simulink model "practica5_simulink"  (R2024b)
settings: Solver=VariableStepAuto  StartTime=0.0  StopTime=0.01  RelTol=1e-3

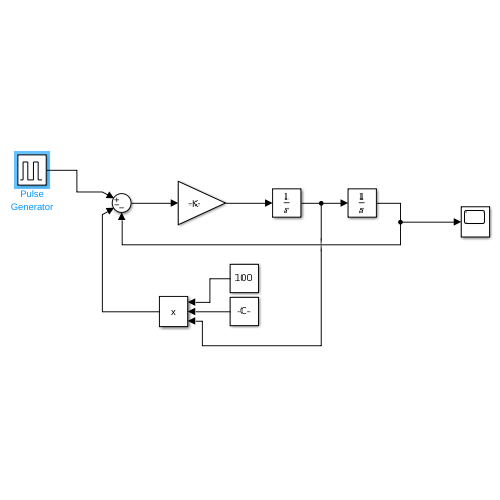
[thumbnail: Simulink's stored preview of the top-level diagram]
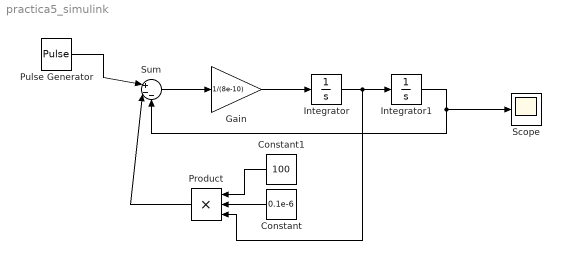
== system practica5_simulink ==
  Constant : Constant  Value=0.1e-6
  Constant1 : Constant  Value=100
  Gain : Gain  Gain=1/(8e-10)
  Integrator : Integrator
  Integrator1 : Integrator
  Product : Product  Inputs=3
  Pulse Generator : DiscretePulseGenerator  PulseType=Time based  Period=0.002  PulseWidth=50
  Scope : Scope
  Sum : Sum  Inputs=|+--
  wires:
  Integrator/1 -> Product/3, Integrator1/1
  Sum/1 -> Gain/1
  Pulse Generator/1 -> Sum/1
  Constant/1 -> Product/2
  Constant1/1 -> Product/1
  Product/1 -> Sum/2
  Integrator1/1 -> Scope/1, Sum/3
  Gain/1 -> Integrator/1
